simulink model ""  (R2018a)
settings: Solver=VariableStepAuto  StartTime=0.0  StopTime=10.0  RelTol=1e-3
settings Model: Creator=rjc1gr  LastModifiedBy=rjc1gr

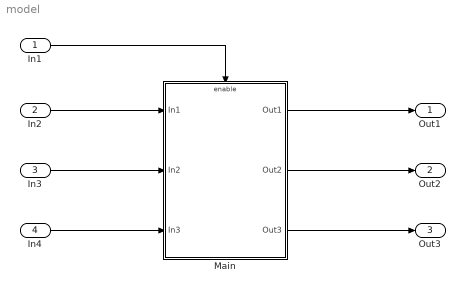
== system model ==
  In1 : Inport
  In2 : Inport  Port=2
  In3 : Inport  Port=3
  In4 : Inport  Port=4
  Main : Subsystem
  Out1 : Outport
  Out2 : Outport  Port=2
  Out3 : Outport  Port=3
  wires:
  In1/1 -> Main/Enable
  In2/1 -> Main/1(In1)
  Main/1(Out1) -> Out1/1
  In4/1 -> Main/3(In3)
  Main/2(Out2) -> Out2/1
  Main/3(Out3) -> Out3/1
  In3/1 -> Main/2(In2)

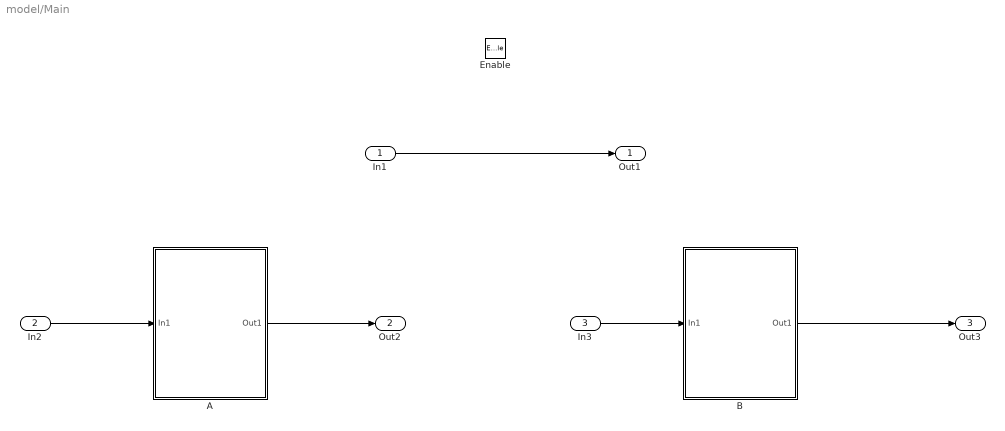
== system model/Main ==
  In1 : Inport
  In2 : Inport  Port=2
  In3 : Inport  Port=3
  Enable : EnablePort
  A : Subsystem
  B : Subsystem
  Out1 : Outport
  Out2 : Outport  Port=2
  Out3 : Outport  Port=3
  wires:
  In1/1 -> Out1/1
  In2/1 -> A/1(In1)
  A/1(Out1) -> Out2/1
  In3/1 -> B/1(In1)
  B/1(Out1) -> Out3/1

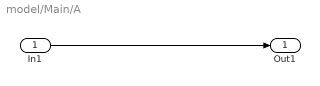
== system model/Main/A ==
  In1 : Inport
  Out1 : Outport
  wires:
  In1/1 -> Out1/1

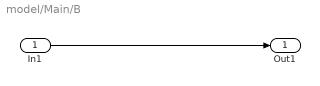
== system model/Main/B ==
  In1 : Inport
  Out1 : Outport
  wires:
  In1/1 -> Out1/1
